simulink model "Sterowanie_slizgowe"  (R2018a)
settings: Solver=VariableStepAuto  StartTime=0.0  StopTime=100  RelTol=1e-3
settings Model: Creator=Szwank  LastModifiedBy=Szwank

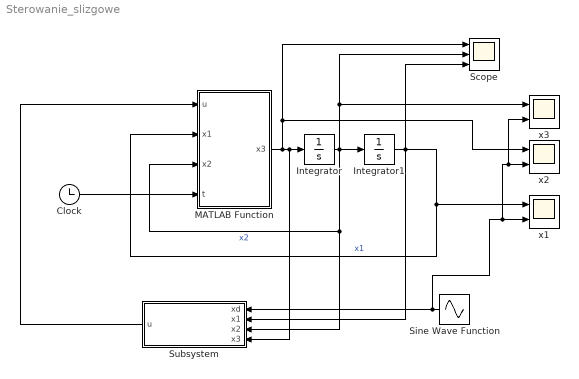
== system Sterowanie_slizgowe ==
  Clock : Clock
  Integrator : Integrator
  Integrator1 : Integrator
  MATLAB Function : MATLAB Function  TreatAsAtomicUnit=on
  Scope : Scope  NumInputPorts=3
  Sine Wave Function : Sin  Frequency=pi/2  SampleTime=1/1000
  Subsystem : Subsystem
  x1 : Scope  NumInputPorts=2
  x2 : Scope  NumInputPorts=2
  x3 : Scope  NumInputPorts=2
  wires:
  MATLAB Function/1(x3) -> x2/1, Scope/1, Subsystem/4(x3), Integrator/1
  Integrator/1 -> x3/1, Scope/2, Subsystem/3(x2), MATLAB Function/3(x2), Integrator1/1  "x2"
  Integrator1/1 -> Subsystem/2(x1), Scope/3, x1/1, MATLAB Function/2(x1)  "x1"
  Clock/1 -> MATLAB Function/4(t)
  Sine Wave Function/1 -> x3/2, x2/2, x1/2, Subsystem/1(xd)
  Subsystem/1(u) -> MATLAB Function/1(u)

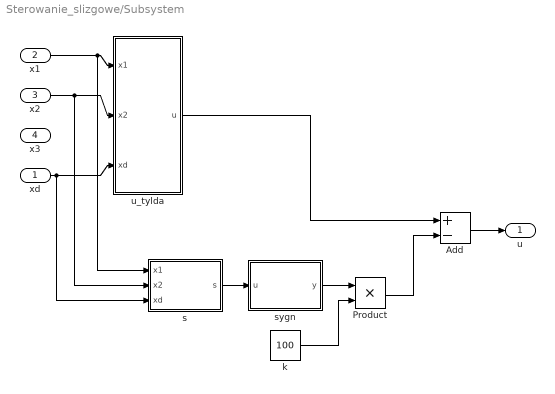
== system Sterowanie_slizgowe/Subsystem ==
  xd : Inport
  x1 : Inport  Port=2  SampleTime=1.0e-03
  x2 : Inport  Port=3  SampleTime=1.0e-03
  x3 : Inport  Port=4  SampleTime=1.0e-03
  Add : Sum  Inputs=+-
  Product : Product
  k : Constant  Value=100
  s : MATLAB Function  TreatAsAtomicUnit=on
  sygn : MATLAB Function  TreatAsAtomicUnit=on
  u_tylda : MATLAB Function  TreatAsAtomicUnit=on
  u : Outport
  wires:
  x1/1 -> s/1(x1), u_tylda/1(x1)
  x2/1 -> s/2(x2), u_tylda/2(x2)
  xd/1 -> s/3(xd), u_tylda/3(xd)
  s/1(s) -> sygn/1(u)
  sygn/1(y) -> Product/1
  k/1 -> Product/2
  Product/1 -> Add/2
  u_tylda/1(u) -> Add/1
  Add/1 -> u/1

== matlab function Sterowanie_slizgowe/Subsystem/u_tylda ==
  data: x1 input; u output; x2 input; xd input
function u = fcn(x1,x2,xd)
%% DANE
alfa = 1.5;
lambda = 300;

%% OBLICZENIA
u = alfa * x2^2 * cos(3*x1) + 0 - lambda * (x2 - 0);

== matlab function Sterowanie_slizgowe/MATLAB Function ==
  data: u input; x3 output; x1 input; x2 input; t input
function x3 = fcn(u,x1,x2,t)
alfa = abs(sin(t)) + 1;
x3 = -alfa * x2^2 * cos(3*x1) + u;

== matlab function Sterowanie_slizgowe/Subsystem/sygn ==
  data: u input; y output
function y = fcn(u)

if u > 0
y = 1;
elseif u < 0 
y = -1;
else 
y = 0;
end

== matlab function Sterowanie_slizgowe/Subsystem/s ==
  data: x1 input; s output; x2 input; xd input
function s = fcn(x1,x2,xd)
lambda = 300;

s = x2-0 + lambda*(x1-xd);
